simulink library "CalibratedSignalBtc"  (R2022b)
settings: Solver=VariableStepAuto  StartTime=0.0  StopTime=10.0  RelTol=1e-3
undefined symbols (not defined in the file or in its folder): Row
libraries: TuneVar x4, HandyTextFile x2, TOP x2, FeaturePath x1, RTC x1
settings Model: Creator=kl13806  LastModifiedBy=kl13806
settings SolverCC: AlgebraicLoopSolver=TrustRegion
settings DebuggingCC: UnconnectedInputMsg=warning  UnconnectedOutputMsg=warning  UnconnectedLineMsg=warning  SFMachineParentedDataDiag=warning
settings ModelReferenceCC: EnableRefExpFcnMdlSchedulingChecks=on
settings RTWCC: DLArmComputeVersion=19.05

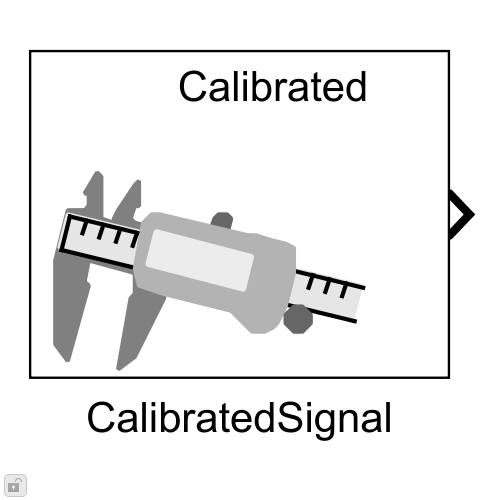
[thumbnail: Simulink's stored preview of the top-level diagram]
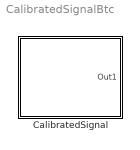
== system CalibratedSignalBtc ==
  CalibratedSignal : Subsystem  mask(Blocklib CalibratedSignal){Config=[], FeatureName=, TriggerInit=[65 26 165 104]}
      mask prompts: Config "CalibratedSignalConfig"; FeatureName "Feature path name:"; TriggerInit "Hidden: MoveFcn redraw"
      mask help: This calibrated signal block sets up runtime receipt of a signal (via RTC) as well as scale and offset tuning variables to calibrate the signal.
      mask init:
      | blkh=gcbh;
      | Config=BTConfig.Assert(blkh,Config);
      | 
      | BTConfig.InitSetFeatureIfPresent(blkh,'FeatureName');
      | Config.Validate();
      | 
      | CalibratedSignalMask.DoInit(blkh,Config);
      settings: MoveFcn=CalibratedSignalMask.CB_TriggerInit(gcbh);
      mask Callback Config: BTConfig.CallbackHideIfPresent(gcbh,{'FeatureName'});
      mask TypeOptions FeatureName: FeaturePath/FeatureName
      mask Callback TriggerInit: CalibratedSignalMask.CB_TriggerInit(gcbh);
      mask Display:
      | [path,w,h] = IconCalibratedSignalMask();
      | 
      | % work in pixels since the icon does not scale
      | pos = get(gcbh,'position');
      | bw = pos(3) - pos(1);
      | bh = pos(4) - pos(2);
      | 
      | % Draw centered icon
      | xAdj = bw/2 - w/2 - 8;
      | yAdj = 2; %bh/2 - h/2 + 4;
      | for i=1:length(path)
      |     if (path(i).rgb(1) >= 0)
      |         patch(path(i).x+xAdj, path(i).y+yAdj, path(i).rgb);
      |     end
      |     if (path(i).stroke(1) >= 0)
      |         plot(path(i).x+xAdj, path(i).y+yAdj);
      |     end
      | end
      | 
      | % Display some text
      | text(bw/2+8, bh-2,['Calibrated\n' FeatureName], ...
      |     'horizontalAlignment','center', ...
      |     'VerticalAlignment','top');

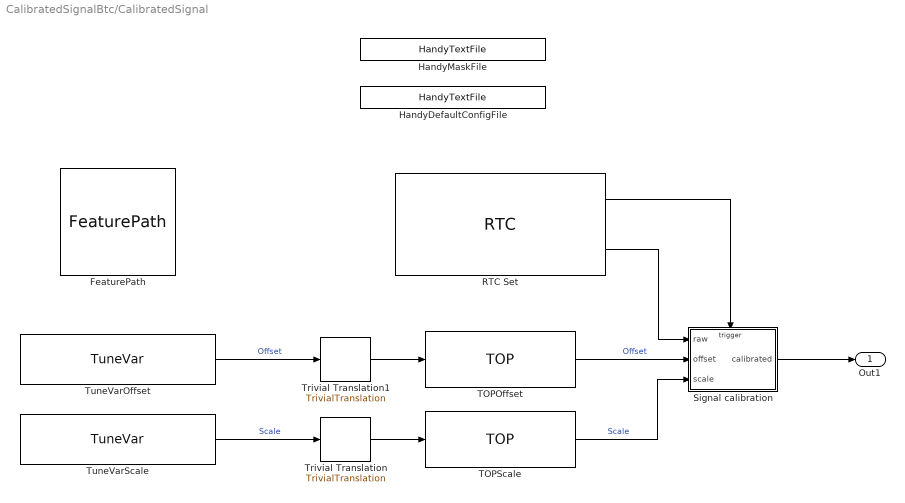
== system CalibratedSignalBtc/CalibratedSignal ==
  FeaturePath : FeaturePath/FeaturePath  IsGroup=off  GroupNumber=-1  IsModule=off  TriggerInit=[260 384 375 491]
      settings: SourceProductName=Bose Talaria
  HandyDefaultConfigFile : HandyTextFile/HandyTextFile  TemplateSource=Config  FileSuffix=Init  OpenDialogOnLoad=off  UseThisBlockName=off  AddGrandParentNamePrefix=off  TheDefaultText=|  ShowInLibBrowser=on
      | % $(FILENAME) Setup model parameters for each "Init" callback (e.g. update diagram)
      | sample_rate_in_hertz = 44100;
      | frame_size = 32;
      | sysin_channel_count = 2;
      settings: SourceProductName=Bose Talaria
  HandyMaskFile : HandyTextFile/HandyTextFile  TemplateSource=<dialog fields>  FileSuffix=Mask  OpenDialogOnLoad=off  UseThisBlockName=off  AddGrandParentNamePrefix=off  TheDefaultText=|  ShowInLibBrowser=on
      | % $(FILENAME) Setup model parameters for each "Init" callback (e.g. update diagram)
      | sample_rate_in_hertz = 44100;
      | frame_size = 32;
      | sysin_channel_count = 2;
      settings: SourceProductName=Bose Talaria
  RTC Set : RTC/RTC  Description=Receives signal as a raw value straight from an external source such as a vehicle network. The tunable variables Scale and Offset are intended to transform the raw value into the units desired by the DSP algorithm. No response or notification is provided to the receipt of the raw vehicle signal.  REQ_Priority=RTC_Mask.HighPriority  RequestAtInit=off  EnableRequest=on  REQElemName1=raw_signal  REQElemType1=uint32  REQElemWidth1=1  REQElemInitial1=[]  REQElemType2=uint32  REQElemWidth2=1  REQElemInitial2=[]  REQElemType3=uint32  REQElemWidth3=1  REQElemInitial3=[]  REQElemType4=uint32  REQElemWidth4=1  REQElemInitial4=[]  REQElemType5=uint32  REQElemWidth5=1  REQElemInitial5=[]  REQElemType6=uint32  REQElemWidth6=1  REQElemInitial6=[]  REQElemType7=uint32  REQElemWidth7=1  REQElemInitial7=[]  REQElemType8=uint32  REQElemWidth8=1  REQElemInitial8=[]  REQElemType9=uint32  REQElemWidth9=1  REQElemInitial9=[]  REQElemType10=uint32  REQElemWidth10=1  REQElemInitial10=[]  EnableResponse=off  EnableRSP_StatusIn=off  RSPElemType1=uint32  RSPElemWidth1=1  RSPElemType2=uint32  RSPElemWidth2=1  RSPElemType3=uint32  RSPElemWidth3=1  RSPElemType4=uint32  RSPElemWidth4=1  RSPElemType5=uint32  RSPElemWidth5=1  RSPElemType6=uint32  RSPElemWidth6=1  RSPElemType7=uint32  RSPElemWidth7=1  RSPElemType8=uint32  RSPElemWidth8=1  RSPElemType9=uint32  RSPElemWidth9=1  RSPElemType10=uint32  RSPElemWidth10=1  EnableNotification=off  EnableNTF_PrepTrig=off  NTFElemType1=uint32  NTFElemWidth1=1  NTFElemType2=uint32  NTFElemWidth2=1  NTFElemType3=uint32  NTFElemWidth3=1  NTFElemType4=uint32  NTFElemWidth4=1  NTFElemType5=uint32  NTFElemWidth5=1  NTFElemType6=uint32  NTFElemWidth6=1  NTFElemType7=uint32  NTFElemWidth7=1  NTFElemType8=uint32  NTFElemWidth8=1  NTFElemType9=uint32  NTFElemWidth9=1  NTFElemType10=uint32  NTFElemWidth10=1  MaskMessageName=Set
      settings: SourceProductName=Bose Talaria
  Signal calibration : Subsystem
  TOPOffset : TOP/TOP  TriggerInit=[625 547 775 603]  TopName=Offset  DataType=Inherit: Same as input  BankNumber=Config.BankNumber  PreOverlay=false  PostOverlay=false  Role=Automatic
      settings: SourceProductName=Bose Talaria
  TOPScale : TOP/TOP  TriggerInit=[625 627 775 683]  TopName=Scale  DataType=Inherit: Same as input  BankNumber=Config.BankNumber  PreOverlay=false  PostOverlay=false  Role=Automatic
      settings: SourceProductName=Bose Talaria
  Trivial Translation : TuneVar/TrivialTranslation  TriggerInit=[520 633 570 677]
      settings: SourceProductName=Bose Talaria
  Trivial Translation1 : TuneVar/TrivialTranslation  TriggerInit=[520 553 570 597]
      settings: SourceProductName=Bose Talaria
  TuneVarOffset : TuneVar/TuneVar  Description=|  TuneName=Offset  SpecifyMaxSize=off  VariableDim=1 (Row)  MaxSize=[1 1]  TunabilityNumber=2  MinValue=[]  MaxValue=[]  TriggerInit=[220 550 415 600]  MaskValue=Config.DefaultOffset
      | Signal calibration.
      | Set Scale and Offset so the following equation becomes true:
      | target-algorithm-signal = (raw-vehicle-signal + Offset)  * Scale
      settings: SourceProductName=Bose Talaria
  TuneVarScale : TuneVar/TuneVar  Description=|  TuneName=Scale  SpecifyMaxSize=off  VariableDim=1 (Row)  MaxSize=[1 1]  TunabilityNumber=2  MinValue=[]  MaxValue=[]  TriggerInit=[220 630 415 680]  MaskValue=Config.DefaultScale
      | Signal calibration.
      | Set Scale and Offset so the following equation becomes true:
      | target-algorithm-signal = (raw-vehicle-signal + Offset)  * Scale
      settings: SourceProductName=Bose Talaria
  Out1 : Outport  VectorParamsAs1DForOutWhenUnconnected=off
  wires:
  RTC Set/1 -> Signal calibration/Trigger
  TOPOffset/1 -> Signal calibration/2(offset)  "Offset"
  TOPScale/1 -> Signal calibration/3(scale)  "Scale"
  RTC Set/2 -> Signal calibration/1(raw)
  Trivial Translation1/1 -> TOPOffset/1
  Trivial Translation/1 -> TOPScale/1
  TuneVarOffset/1 -> Trivial Translation1/1  "Offset"
  TuneVarScale/1 -> Trivial Translation/1  "Scale"
  Signal calibration/1(calibrated) -> Out1/1

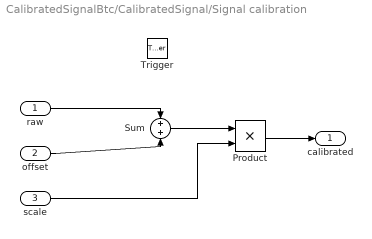
== system CalibratedSignalBtc/CalibratedSignal/Signal calibration ==
  raw : Inport
  offset : Inport  Port=2
  scale : Inport  Port=3
  Trigger : TriggerPort  TriggerType=function-call  VariantControl=Variant  PortDimensions=1
  Product : Product  LockScale=on
  Sum : Sum
  calibrated : Outport  VectorParamsAs1DForOutWhenUnconnected=off
  wires:
  raw/1 -> Sum/1
  Sum/1 -> Product/1
  Product/1 -> calibrated/1
  offset/1 -> Sum/2
  scale/1 -> Product/2
